simulink model "Ex1_1"  (R2021b)
settings: Solver=VariableStepAuto  StartTime=0.0  StopTime=10.0  RelTol=1e-3
values from neighbouring files (symbols this model uses):
  C = 1e-3    (= 0.001)    [Ex1_1_comp.m]
  R = [100;1e3]    [Ex1_1_comp.m]
settings Model: Creator=gaeta  LastModifiedBy=gaeta

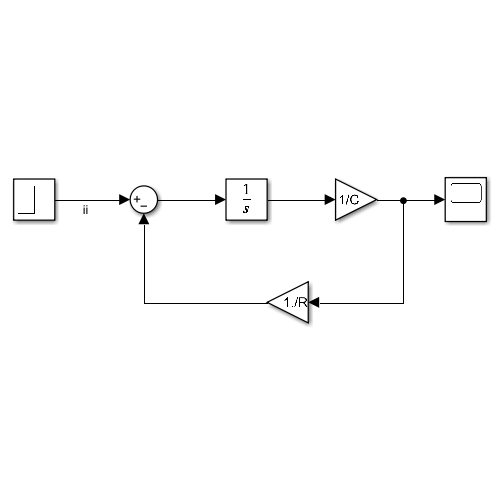
[thumbnail: Simulink's stored preview of the top-level diagram]
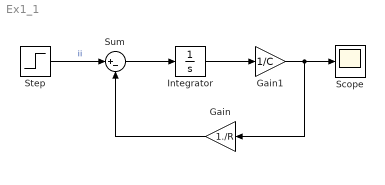
== system Ex1_1 ==
  Gain : Gain  Gain=1./R
  Gain1 : Gain  Gain=1/C
  Integrator : Integrator
  Scope : Scope
  Step : Step  SampleTime=0
  Sum : Sum  Inputs=|+-
  wires:
  Step/1 -> Sum/1  "ii"
  Sum/1 -> Integrator/1
  Gain/1 -> Sum/2
  Integrator/1 -> Gain1/1
  Gain1/1 -> Gain/1, Scope/1
